simulink model "xdot_obac_debug"  (Simulink 6.3)
settings: Solver=FixedStepDiscrete  StartTime=0.0  StopTime=0  RelTol=1e-3
undefined symbols (not defined in the file or in its folder): aero, bspan, cbar, constants, Frcs, MACH, MACH_mass_IC, obac_params, r_aero, r_prop, r_rcs, rcs_idx, Sref, throt_to_ff, tvc_idx
libraries: simulink x14, models x14, utility_lib x12, model_lib x3, aerospace x1
settings Model: LastModifiedBy=E700252  BufferReuse=off  StrictBusMsg=None
settings DataIOCC: ExternalInput=[0 xu]  InitialState=[]  LoadExternalInput=on  LoadInitialState=on  SaveOutput=off  SaveTime=off  SignalLoggingName=sigsOut
settings OptimizationCC: InlineParams=on  BufferReuse=off
settings DebuggingCC: SolverPrmCheckMsg=none
settings HardwareCC: TargetUnknown=on

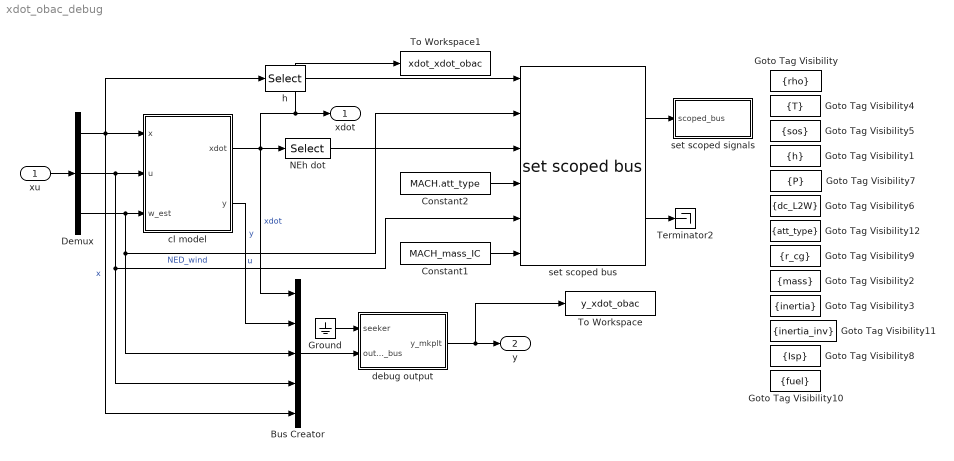
== system xdot_obac_debug ==
  xu : Inport
  Bus Creator : BusCreator  Inputs=5
  Constant1 : Constant  Value=MACH_mass_IC
  Constant2 : Constant  Value=MACH.att_type
  Demux : Demux  Outputs=[MACH.num_x MACH.num_u 3]
  Goto Tag Visibility : GotoTagVisibility  GotoTag=rho
  Goto Tag Visibility1 : GotoTagVisibility  GotoTag=h
  Goto Tag Visibility10 : GotoTagVisibility  GotoTag=fuel
  Goto Tag Visibility11 : GotoTagVisibility  GotoTag=inertia_inv
  Goto Tag Visibility12 : GotoTagVisibility  GotoTag=att_type
  Goto Tag Visibility2 : GotoTagVisibility  GotoTag=mass
  Goto Tag Visibility3 : GotoTagVisibility  GotoTag=inertia
  Goto Tag Visibility4 : GotoTagVisibility  GotoTag=T
  Goto Tag Visibility5 : GotoTagVisibility  GotoTag=sos
  Goto Tag Visibility6 : GotoTagVisibility  GotoTag=dc_L2W
  Goto Tag Visibility7 : GotoTagVisibility  GotoTag=P
  Goto Tag Visibility8 : GotoTagVisibility  GotoTag=Isp
  Goto Tag Visibility9 : GotoTagVisibility  GotoTag=r_cg
  Ground : Ground
  NEh dot : Selector  Elements=MACH.NEh_idx  InputPortWidth=obac_params.num_x
  Terminator2 : Terminator
  To Workspace : ToWorkspace  VariableName=y_xdot_obac  SampleTime=-1  SaveFormat=Array
  To Workspace1 : ToWorkspace  VariableName=xdot_xdot_obac  SampleTime=-1  SaveFormat=Array
  cl model : Subsystem  AncestorBlock=models/datcom-obac
  debug output : Subsystem
  h : Selector  Elements=MACH.NEh_idx(3)  InputPortWidth=obac_params.num_x
  set scoped bus : model_lib/set scoped bus  vehicle_params=obac_params
  set scoped signals : Subsystem  AncestorBlock=model_lib/set scoped signals
  xdot : Outport
  y : Outport  Port=2
  wires:
  Demux/1 -> cl model/1(x), h/1, Bus Creator/5  "x"
  Demux/2 -> cl model/2(u), set scoped bus/5, Bus Creator/4  "u"
  Demux/3 -> cl model/3(w_est), set scoped bus/2, Bus Creator/3  "NED_wind"
  xu/1 -> Demux/1
  cl model/1(xdot) -> NEh dot/1, Bus Creator/1, xdot/1, To Workspace1/1  "xdot"
  h/1 -> set scoped bus/1
  NEh dot/1 -> set scoped bus/3
  Constant2/1 -> set scoped bus/4
  set scoped bus/1 -> set scoped signals/1(scoped_bus)
  Constant1/1 -> set scoped bus/6
  set scoped bus/2 -> Terminator2/1
  debug output/1(y_mkplt) -> y/1, To Workspace/1
  Ground/1 -> debug output/1(seeker)
  Bus Creator/1 -> debug output/2(output_bus)
  cl model/2(y) -> Bus Creator/2  "y"

== system xdot_obac_debug/cl model ==
  x : Inport
  u : Inport  Port=2
  w_est : Inport  Port=3
  datcom-kernel : Subsystem  AncestorBlock=models/datcom-kernel  mask{vehicle_params=obac_params}
      mask prompts: vehicle_params "vehicle params"
      mask init:
      | paramnames = fieldnames(vehicle_params);
      | for i=1:length(paramnames)
      | 	eval([paramnames{i} '= vehicle_params.' paramnames{i} ';']);
      | end
  xdot : Outport
  y : Outport  Port=2
  wires:
  datcom-kernel/2(y) -> y/1
  datcom-kernel/1(xdot) -> xdot/1
  w_est/1 -> datcom-kernel/3(w_est)
  u/1 -> datcom-kernel/2(u)
  x/1 -> datcom-kernel/1(x)

== system xdot_obac_debug/debug output ==
  seeker : Inport
  output_bus : Inport  Port=2
  Bus Creator1 : BusCreator  Inputs=7
  Bus Selector : BusSelector  OutputSignals=y.dircos,x,NED_wind
  Gain : Gain  SaturateOnIntegerOverflow=on
  angles : Subsystem
  order outputs as expected by mkplt : BusSelector  OutputSignals=output_bus.y.accels,output_bus.y.accels_cg,output_bus.y.dircos,uvw_rw,tilta;tiltb;cam,phi;theta;psi,mu;alpha;beta,mass,output_bus.y.aero_env,seeker  OutputAsBus=on
  uvw : Selector  Elements=MACH.uvw_idx  InputPortWidth=MACH.num_x
  y_mkplt : Outport
  wires:
  Bus Selector/2 -> uvw/1  "<x>"
  Bus Creator1/1 -> order outputs as expected by mkplt/1
  Bus Selector/3 -> angles/3(NED_wind)  "<NED_wind>"
  uvw/1 -> angles/2(uvw)
  Bus Selector/1 -> angles/1(dircos)  "<dircos>"
  seeker/1 -> Bus Creator1/7  "seeker"
  [mass] -> Bus Creator1/6  "mass"
  Gain/1 -> y_mkplt/1
  order outputs as expected by mkplt/1 -> Gain/1
  output_bus/1 -> Bus Creator1/1, Bus Selector/1  "output_bus"
  angles/3(phi;theta;psi) -> Bus Creator1/4  "phi;theta;psi"
  angles/2(tilta;tiltb;cam) -> Bus Creator1/3  "tilta;tiltb;cam"
  angles/1(uvw_rw) -> Bus Creator1/2  "uvw_rw"
  angles/4(mu;alpha;beta) -> Bus Creator1/5  "mu;alpha;beta"

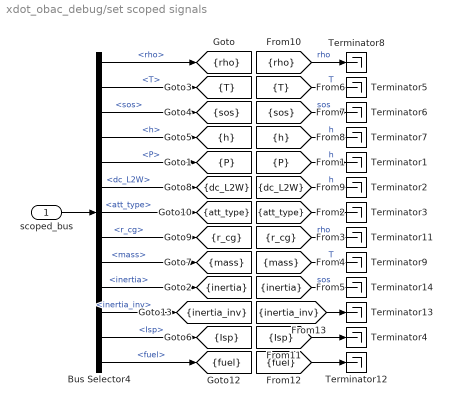
== system xdot_obac_debug/set scoped signals ==
  scoped_bus : Inport
  Bus Selector4 : BusSelector  OutputSignals=atmos_env.rho,atmos_env.T,atmos_env.sos,atmos_env.h,atmos_env.P,dc_L2W,att_type,mass_props.r_cg,mass_props.mass,mass_props.inertia,mass_props.inertia_inv,mass_props.Isp,mass_props.fuel
  Terminator{1..9,11..14} (13 alike) : Terminator
  tag scope: Isp=scoped, P=scoped, T=scoped, att_type=scoped, dc_L2W=scoped, fuel=scoped, h=scoped, inertia=scoped, inertia_inv=scoped, mass=scoped, r_cg=scoped, rho=scoped, sos=scoped
  wires:
  scoped_bus/1 -> Bus Selector4/1
  Bus Selector4/1 -> [rho]  "<rho>"
  Bus Selector4/2 -> [T]  "<T>"
  Bus Selector4/3 -> [sos]  "<sos>"
  Bus Selector4/4 -> [h]  "<h>"
  Bus Selector4/5 -> [P]  "<P>"
  Bus Selector4/6 -> [dc_L2W]  "<dc_L2W>"
  Bus Selector4/7 -> [att_type]  "<att_type>"
  Bus Selector4/8 -> [r_cg]  "<r_cg>"
  Bus Selector4/9 -> [mass]  "<mass>"
  Bus Selector4/10 -> [inertia]  "<inertia>"
  Bus Selector4/12 -> [Isp]  "<Isp>"
  [h] -> Terminator7/1  "h"
  [sos] -> Terminator6/1  "sos"
  [T] -> Terminator5/1  "T"
  [rho] -> Terminator8/1  "rho"
  [P] -> Terminator1/1  "h"
  [dc_L2W] -> Terminator2/1  "h"
  [att_type] -> Terminator3/1
  [r_cg] -> Terminator11/1  "rho"
  [mass] -> Terminator9/1  "T"
  [inertia] -> Terminator14/1  "sos"
  [Isp] -> Terminator4/1
  Bus Selector4/13 -> [fuel]  "<fuel>"
  [fuel] -> Terminator12/1
  [inertia_inv] -> Terminator13/1
  Bus Selector4/11 -> [inertia_inv]  "<inertia_inv>"

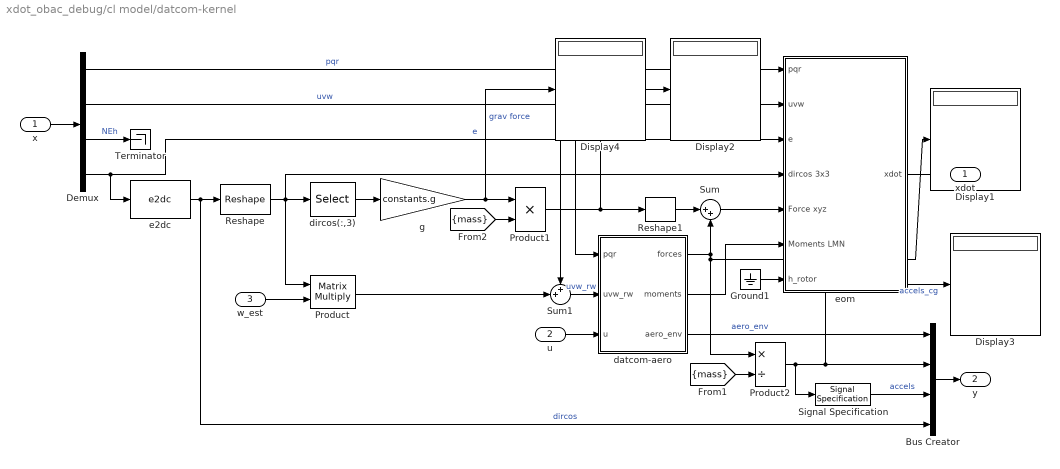
== system xdot_obac_debug/cl model/datcom-kernel ==
  x : Inport
  u : Inport  Port=2
  w_est : Inport  Port=3
  Bus Creator : BusCreator
  Demux : Demux  Outputs=[3 3 3 4]
  Display{1..4} (4 alike) : Display
  Ground1 : Ground
  Product : Product  Multiplication=Matrix(*)  SaturateOnIntegerOverflow=on
  Product1 : Product  RndMeth=Zero
  Product2 : Product  Inputs=*/  RndMeth=Zero
  Reshape : simulink/Math Operations/Reshape  OutputDimensionality=Customize  OutputDimensions=[3,3]
  Reshape1 : simulink/Math Operations/Reshape  OutputDimensionality=1-D array  OutputDimensions=[1,1]
  Signal Specification : SignalSpecification
  Sum : Sum  Inputs=|++  SaturateOnIntegerOverflow=on
  Sum1 : Sum  Inputs=++|  SaturateOnIntegerOverflow=on
  Terminator : Terminator
  datcom-aero : Subsystem  AncestorBlock=models/datcom-aero  mask{aero_params=aero}
      mask prompts: aero_params "aero params"
      mask init:
      | paramnames = fieldnames(aero_params);
      | for i=1:length(paramnames)
      | 	eval([paramnames{i} '= aero_params.' paramnames{i} ';']);
      | end
  dircos(:,3) : Selector  InputType=Matrix  Elements=[7:9]  Rows=-1  Columns=3  InputPortWidth=9
  e2dc : utility_lib/e2dc
  eom : Subsystem  AncestorBlock=model_lib/eom
  g : Gain  Gain=constants.g  SaturateOnIntegerOverflow=on
  xdot : Outport
  y : Outport  Port=2
  wires:
  Signal Specification/1 -> Bus Creator/3  "accels"
  Bus Creator/1 -> y/1
  [mass] -> Product2/2
  Product2/1 -> Signal Specification/1, Bus Creator/2, Display3/1  "accels_cg"
  x/1 -> Demux/1
  Demux/1 -> datcom-aero/1(pqr), eom/1(pqr)  "pqr"
  Demux/3 -> Terminator/1  "NEh"
  Demux/4 -> eom/3(e), e2dc/1  "e"
  Demux/2 -> eom/2(uvw), Sum1/1  "uvw"
  dircos(:,3)/1 -> g/1
  g/1 -> Product1/1, Display4/1  "grav force"
  eom/1(xdot) -> xdot/1
  e2dc/1 -> Bus Creator/4, Reshape/1  "dircos"
  u/1 -> datcom-aero/3(u)
  datcom-aero/1(forces) -> Sum/2, Product2/1, Display1/1
  Sum1/1 -> datcom-aero/2(uvw_rw)  "uvw_rw"
  w_est/1 -> Product/2
  Product/1 -> Sum1/2
  Sum/1 -> eom/5("Force xyz ")
  Reshape/1 -> eom/4(dircos 3x3), dircos(:,3)/1, Product/1
  Reshape1/1 -> Sum/1
  datcom-aero/2(moments) -> eom/6(Moments LMN)
  Ground1/1 -> eom/7(h_rotor)
  datcom-aero/3(aero_env) -> Bus Creator/1  "aero_env"
  Product1/1 -> Reshape1/1, Display2/1
  [mass] -> Product1/2

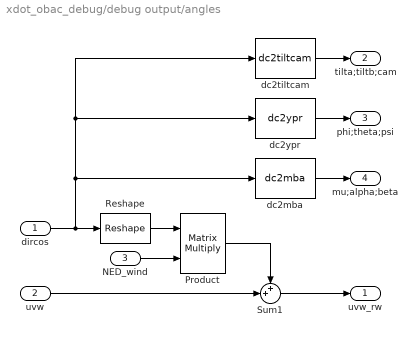
== system xdot_obac_debug/debug output/angles ==
  dircos : Inport
  uvw : Inport  Port=2
  NED_wind : Inport  Port=3
  Product : Product  Multiplication=Matrix(*)  SaturateOnIntegerOverflow=on
  Reshape : simulink/Math Operations/Reshape  OutputDimensionality=Customize  OutputDimensions=[3,3]
  Sum1 : Sum  Inputs=++|  SaturateOnIntegerOverflow=on
  dc2mba : utility_lib/dc2mba
  dc2tiltcam : utility_lib/dc2tiltcam
  dc2ypr : utility_lib/dc2ypr
  uvw_rw : Outport
  tilta;tiltb;cam : Outport  Port=2
  phi;theta;psi : Outport  Port=3
  mu;alpha;beta : Outport  Port=4
  wires:
  dircos/1 -> dc2mba/1, dc2tiltcam/1, dc2ypr/1, Reshape/1
  Reshape/1 -> Product/1
  dc2mba/1 -> mu;alpha;beta/1
  dc2tiltcam/1 -> tilta;tiltb;cam/1
  dc2ypr/1 -> phi;theta;psi/1
  Sum1/1 -> uvw_rw/1
  uvw/1 -> Sum1/2
  Product/1 -> Sum1/1
  NED_wind/1 -> Product/2

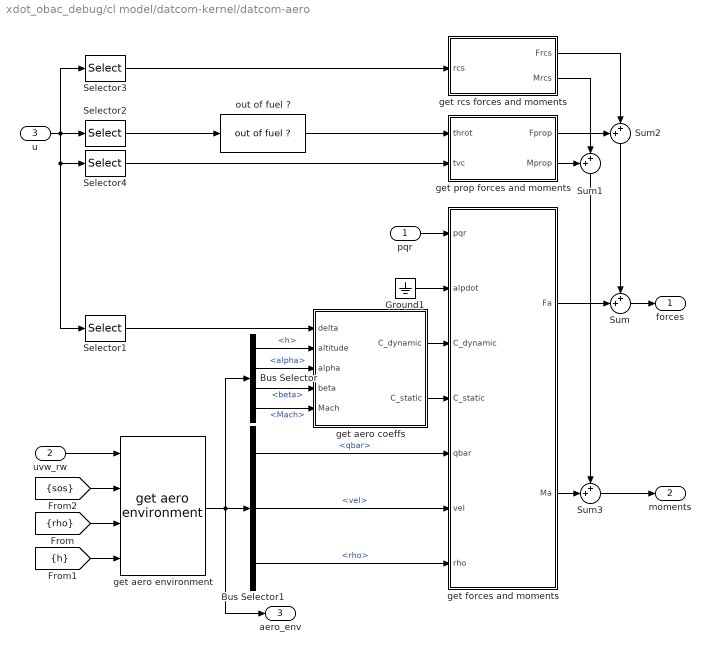
== system xdot_obac_debug/cl model/datcom-kernel/datcom-aero ==
  pqr : Inport
  uvw_rw : Inport  Port=2
  u : Inport  Port=3
  Bus Selector : BusSelector  OutputSignals=h,alpha,beta,Mach
  Bus Selector1 : BusSelector  OutputSignals=qbar,vel,rho
  Ground1 : Ground
  Selector1 : Selector  Elements=vane_idx  InputPortWidth=num_u
  Selector2 : Selector  Elements=throttle_idx  InputPortWidth=num_u
  Selector3 : Selector  Elements=[rcs_idx 1]  InputPortWidth=num_u
  Selector4 : Selector  Elements=tvc_idx  InputPortWidth=num_u
  Sum : Sum  Inputs=++|
  Sum1 : Sum  Orientation=down  Inputs=++|
  Sum2 : Sum  Orientation=down  Inputs=++|
  Sum3 : Sum  Inputs=++|
  get aero coeffs : Subsystem
  get aero environment : model_lib/get aero environment
  get forces and moments : Subsystem
  get prop forces and moments : Subsystem  AncestorBlock=model_lib/get prop forces and moments
  get rcs forces and moments : Subsystem
  out of fuel ? : model_lib/out of fuel ?
  forces : Outport
  moments : Outport  Port=2
  aero_env : Outport  Port=3
  wires:
  [rho] -> get aero environment/3
  pqr/1 -> get forces and moments/1(pqr)
  uvw_rw/1 -> get aero environment/1
  get aero coeffs/1(C_dynamic) -> get forces and moments/3(C_dynamic)
  get aero coeffs/2(C_static) -> get forces and moments/4(C_static)
  Ground1/1 -> get forces and moments/2(alpdot)
  get forces and moments/1(Fa) -> Sum/2
  Selector1/1 -> get aero coeffs/1(delta)
  [sos] -> get aero environment/2
  get aero environment/1 -> Bus Selector/1, Bus Selector1/1, aero_env/1
  Bus Selector/2 -> get aero coeffs/3(alpha)  "<alpha>"
  Bus Selector/3 -> get aero coeffs/4(beta)  "<beta>"
  Bus Selector/4 -> get aero coeffs/5(Mach)  "<Mach>"
  Bus Selector1/1 -> get forces and moments/5(qbar)  "<qbar>"
  Bus Selector1/2 -> get forces and moments/6(vel)  "<vel>"
  Bus Selector/1 -> get aero coeffs/2(altitude)  "<h>"
  [h] -> get aero environment/4
  Bus Selector1/3 -> get forces and moments/7(rho)  "<rho>"
  u/1 -> Selector2/1, Selector3/1, Selector1/1, Selector4/1
  Selector3/1 -> get rcs forces and moments/1(rcs)
  Sum/1 -> forces/1
  Sum3/1 -> moments/1
  get forces and moments/2(Ma) -> Sum3/2
  get rcs forces and moments/1(Frcs) -> Sum2/2
  get rcs forces and moments/2(Mrcs) -> Sum1/2
  get prop forces and moments/2(Mprop) -> Sum1/1
  get prop forces and moments/1(Fprop) -> Sum2/1
  Sum2/1 -> Sum/1
  Sum1/1 -> Sum3/1
  Selector2/1 -> out of fuel ?/1
  Selector4/1 -> get prop forces and moments/2(tvc)
  out of fuel ?/1 -> get prop forces and moments/1(throt)

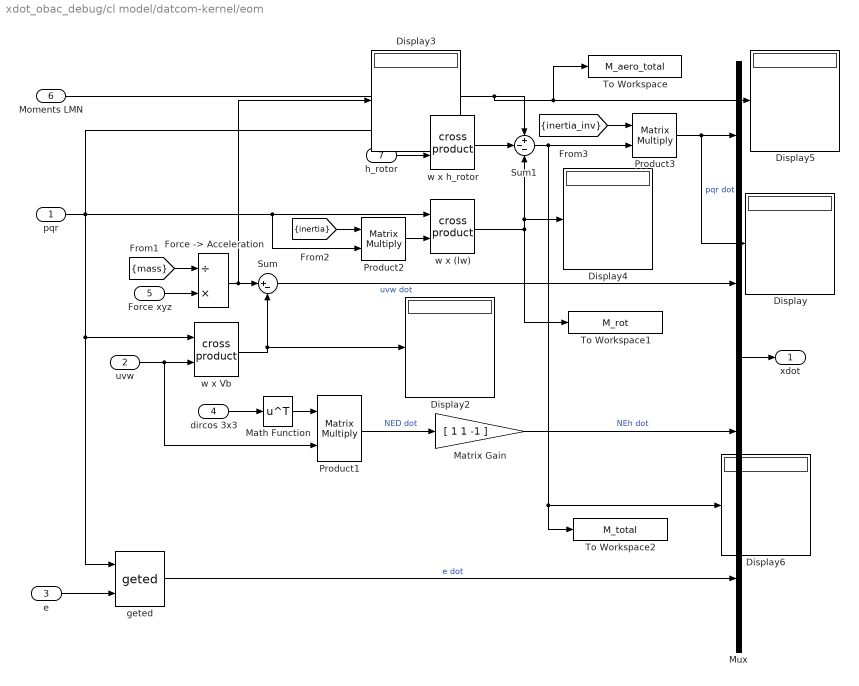
== system xdot_obac_debug/cl model/datcom-kernel/eom ==
  pqr : Inport
  uvw : Inport  Port=2
  e : Inport  Port=3
  dircos 3x3 : Inport  Port=4
  "Force xyz " : Inport  Port=5
  Moments LMN : Inport  Port=6
  h_rotor : Inport  Port=7
  Display{,2..6} (6 alike) : Display
  "Force -> Acceleration" : Product  Inputs=/*  RndMeth=Zero
  Math Function : Math  Operator=transpose  SaturateOnIntegerOverflow=on
  Matrix Gain : Gain  Gain=[ 1 1 -1 ]  SaturateOnIntegerOverflow=on
  Mux : Mux
  Product1 : Product  Multiplication=Matrix(*)  SaturateOnIntegerOverflow=on  InputSameDT=on
  Product2 : Product  Multiplication=Matrix(*)  RndMeth=Zero
  Product3 : Product  Multiplication=Matrix(*)  RndMeth=Zero
  Sum : Sum  Inputs=|+-  SaturateOnIntegerOverflow=on
  Sum1 : Sum  Inputs=+--  SaturateOnIntegerOverflow=on
  To Workspace : ToWorkspace  VariableName=M_aero_total  SampleTime=-1  SaveFormat=Array
  To Workspace1 : ToWorkspace  VariableName=M_rot  SampleTime=-1  SaveFormat=Array
  To Workspace2 : ToWorkspace  VariableName=M_total  SampleTime=-1  SaveFormat=Array
  geted : utility_lib/geted
  w x (lw) : utility_lib/cross product
  w x Vb : utility_lib/cross product
  w x h_rotor : utility_lib/cross product
  xdot : Outport
  wires:
  [inertia_inv] -> Product3/1
  [mass] -> "Force -> Acceleration"/1
  [inertia] -> Product2/1
  w x h_rotor/1 -> Sum1/2
  w x (lw)/1 -> Sum1/3, Display4/1, To Workspace1/1
  h_rotor/1 -> w x h_rotor/2
  "Force -> Acceleration"/1 -> Sum/1, Display3/1
  Math Function/1 -> Product1/1
  Product1/1 -> Matrix Gain/1  "NED dot"
  Sum1/1 -> Product3/2, Display6/1, To Workspace2/1
  Moments LMN/1 -> Sum1/1, Display5/1, To Workspace/1
  Product2/1 -> w x (lw)/2
  Product3/1 -> Mux/1, Display/1  "pqr dot"
  pqr/1 -> w x h_rotor/1, w x (lw)/1, Product2/2, w x Vb/1, geted/1
  dircos 3x3/1 -> Math Function/1
  Matrix Gain/1 -> Mux/3  "NEh dot"
  Sum/1 -> Mux/2  "uvw dot"
  "Force xyz "/1 -> "Force -> Acceleration"/2
  w x Vb/1 -> Sum/2, Display2/1
  uvw/1 -> w x Vb/2, Product1/2
  e/1 -> geted/2
  geted/1 -> Mux/4  "e dot"
  Mux/1 -> xdot/1

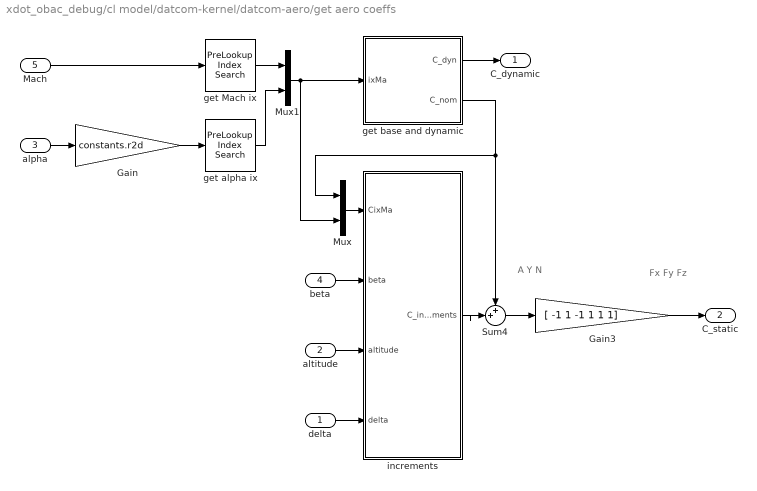
== system xdot_obac_debug/cl model/datcom-kernel/datcom-aero/get aero coeffs ==
  note: A
      | Y
      | N
  note: Fx
      | Fy
      | Fz
  delta : Inport
  altitude : Inport  Port=2
  alpha : Inport  Port=3
  beta : Inport  Port=4
  Mach : Inport  Port=5
  Gain : Gain  Gain=constants.r2d
  Gain3 : Gain  Gain=[ -1 1 -1 1 1 1]
  Mux : Mux  Inputs=2
  Mux1 : Mux  Inputs=2
  Sum4 : Sum  Inputs=++|
  get Mach ix : simulink/Lookup Tables/PreLookup Index Search  bpData=tbl_mach  searchMode=Binary Search  cacheBpFlag=off  outputFlag=off  IndexDataType=uint32  extrapMode=Linear Extrapolation  rangeErrorMode=None
  get alpha ix : simulink/Lookup Tables/PreLookup Index Search  bpData=tbl_alpha  searchMode=Binary Search  cacheBpFlag=off  outputFlag=off  IndexDataType=uint32  extrapMode=Linear Extrapolation  rangeErrorMode=None
  get base and dynamic : Subsystem
  increments : Subsystem
  C_dynamic : Outport
  C_static : Outport  Port=2
  wires:
  Mux1/1 -> get base and dynamic/1(ixMa), Mux/2
  get alpha ix/1 -> Mux1/2
  get Mach ix/1 -> Mux1/1
  alpha/1 -> Gain/1
  beta/1 -> increments/2(beta)
  delta/1 -> increments/4(delta)
  Mach/1 -> get Mach ix/1
  get base and dynamic/2(C_nom) -> Sum4/1, Mux/1
  Sum4/1 -> Gain3/1
  Mux/1 -> increments/1(CixMa)
  altitude/1 -> increments/3(altitude)
  increments/1(C_increments) -> Sum4/2
  get base and dynamic/1(C_dyn) -> C_dynamic/1
  Gain/1 -> get alpha ix/1
  Gain3/1 -> C_static/1

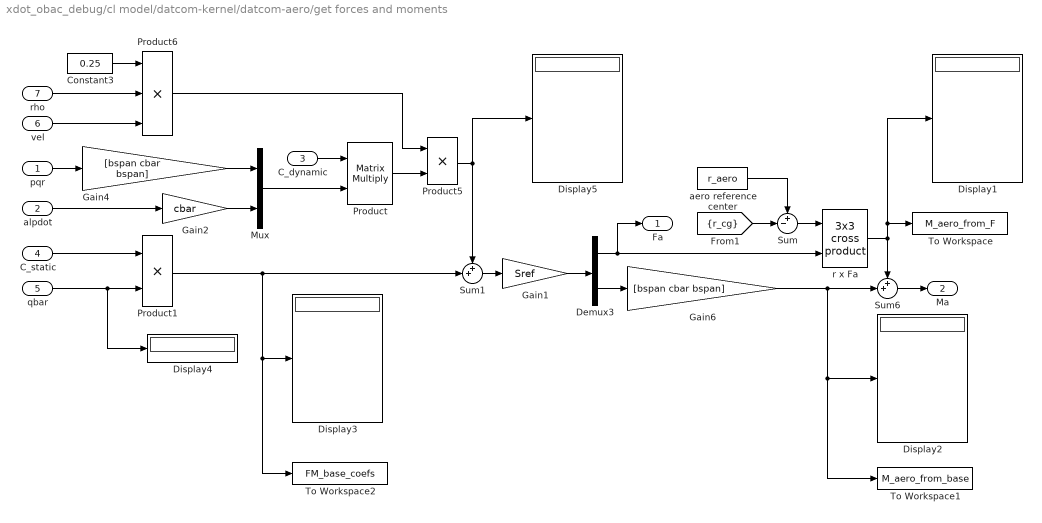
== system xdot_obac_debug/cl model/datcom-kernel/datcom-aero/get forces and moments ==
  pqr : Inport
  alpdot : Inport  Port=2
  C_dynamic : Inport  Port=3
  C_static : Inport  Port=4
  qbar : Inport  Port=5
  vel : Inport  Port=6
  rho : Inport  Port=7
  Constant3 : Constant  Value=0.25
  Demux3 : Demux  Outputs=2
  Display{1..5} (5 alike) : Display
  Gain1 : Gain  Gain=Sref
  Gain2 : Gain  Gain=cbar
  Gain4 : Gain  Gain=[bspan cbar bspan]
  Gain6 : Gain  Gain=[bspan cbar bspan]
  Mux : Mux  Inputs=2
  Product : Product  Multiplication=Matrix(*)  RndMeth=Zero
  Product1 : Product  RndMeth=Zero
  Product5 : Product  RndMeth=Zero
  Product6 : Product  Inputs=3  RndMeth=Zero
  Sum : Sum  Inputs=+-|
  Sum1 : Sum  Inputs=++|
  Sum6 : Sum  Inputs=++|
  To Workspace : ToWorkspace  VariableName=M_aero_from_F  SampleTime=-1  SaveFormat=Array
  To Workspace1 : ToWorkspace  VariableName=M_aero_from_base  SampleTime=-1  SaveFormat=Array
  To Workspace2 : ToWorkspace  VariableName=FM_base_coefs  SampleTime=-1  SaveFormat=Array
  aero reference center : Constant  Value=r_aero
  r x Fa : aerospace/Axes Transformations/3x3 cross product
  Fa : Outport
  Ma : Outport  Port=2
  wires:
  qbar/1 -> Product1/2, Display4/1
  C_static/1 -> Product1/1
  Gain1/1 -> Demux3/1
  Demux3/2 -> Gain6/1
  Demux3/1 -> r x Fa/2, Fa/1
  Sum1/1 -> Gain1/1
  Product/1 -> Product5/2
  Mux/1 -> Product/2
  Gain2/1 -> Mux/2
  Gain4/1 -> Mux/1
  alpdot/1 -> Gain2/1
  r x Fa/1 -> Sum6/1, Display1/1, To Workspace/1
  Sum6/1 -> Ma/1
  Constant3/1 -> Product6/1
  rho/1 -> Product6/2
  vel/1 -> Product6/3
  Product6/1 -> Product5/1
  Product5/1 -> Sum1/1, Display5/1
  Product1/1 -> Sum1/2, Display3/1, To Workspace2/1
  C_dynamic/1 -> Product/1
  pqr/1 -> Gain4/1
  Gain6/1 -> Sum6/2, Display2/1, To Workspace1/1
  aero reference center/1 -> Sum/1
  [r_cg] -> Sum/2
  Sum/1 -> r x Fa/1

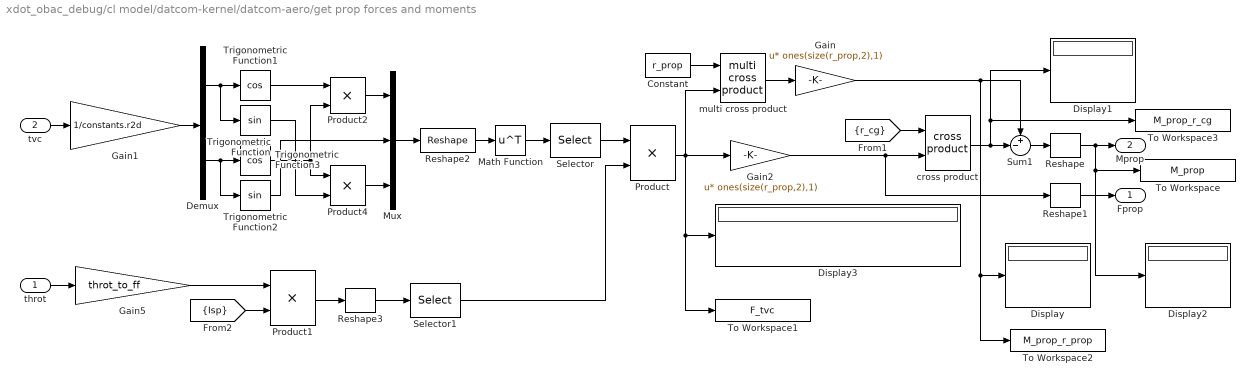
== system xdot_obac_debug/cl model/datcom-kernel/datcom-aero/get prop forces and moments ==
  throt : Inport
  tvc : Inport  Port=2
  Constant : Constant  Value=r_prop  VectorParams1D=off
  Demux : Demux  Outputs=2
  Display{,1..3} (4 alike) : Display
  Gain : Gain  Gain=ones(size(r_prop,2),1)  Multiplication=Matrix(u*K)
  Gain1 : Gain  Gain=1/constants.r2d
  Gain2 : Gain  Gain=ones(size(r_prop,2),1)  Multiplication=Matrix(u*K)
  Gain5 : Gain  Gain=throt_to_ff
  Math Function : Math  Operator=transpose  SaturateOnIntegerOverflow=on
  Mux : Mux  Inputs=3
  Product{,1..2,4} (4 alike) : Product  RndMeth=Zero
  Reshape : simulink/Math Operations/Reshape  OutputDimensionality=1-D array  OutputDimensions=[1,1]
  Reshape1 : simulink/Math Operations/Reshape  OutputDimensionality=1-D array  OutputDimensions=[1,1]
  Reshape2 : simulink/Math Operations/Reshape  OutputDimensionality=Customize  OutputDimensions=[length(tvc_idx)/2 3]
  Reshape3 : simulink/Math Operations/Reshape  OutputDimensionality=Row vector  OutputDimensions=[1,1]
  Selector : Selector  InputType=Matrix  Elements=[1 3]  Rows=-1  Columns=min(1:size(r_prop,2),length(tvc_idx)/2)  InputPortWidth=3
  Selector1 : Selector  InputType=Matrix  Elements=[1 3]  Rows=ones(1,size(r_prop,2))  Columns=-1  InputPortWidth=3
  Sum1 : Sum  Inputs=+-|
  To Workspace : ToWorkspace  VariableName=M_prop  SampleTime=-1  SaveFormat=Array
  To Workspace1 : ToWorkspace  VariableName=F_tvc  SampleTime=-1  SaveFormat=Array
  To Workspace2 : ToWorkspace  VariableName=M_prop_r_prop  SampleTime=-1  SaveFormat=Array
  To Workspace3 : ToWorkspace  VariableName=M_prop_r_cg  SampleTime=-1  SaveFormat=Array
  Trigonometric Function : Trigonometry
  Trigonometric Function1 : Trigonometry  Operator=cos
  Trigonometric Function2 : Trigonometry
  Trigonometric Function3 : Trigonometry  Operator=cos
  cross product : utility_lib/cross product
  multi cross product : utility_lib/multi cross product
  Fprop : Outport
  Mprop : Outport  Port=2
  wires:
  Reshape3/1 -> Selector1/1
  Selector1/1 -> Product/2
  Selector/1 -> Product/1
  Math Function/1 -> Selector/1
  Reshape2/1 -> Math Function/1
  Reshape1/1 -> Fprop/1
  Reshape/1 -> Mprop/1, To Workspace/1, Display2/1
  Sum1/1 -> Reshape/1
  cross product/1 -> Sum1/2, Display1/1, To Workspace3/1
  Gain/1 -> Sum1/1, Display/1, To Workspace2/1
  multi cross product/1 -> Gain/1
  Gain2/1 -> cross product/2, Reshape1/1
  [r_cg] -> cross product/1
  Product/1 -> multi cross product/2, Gain2/1, Display3/1, To Workspace1/1
  Constant/1 -> multi cross product/1
  tvc/1 -> Gain1/1
  Demux/1 -> Trigonometric Function1/1, Trigonometric Function/1
  Demux/2 -> Trigonometric Function3/1, Trigonometric Function2/1
  Product4/1 -> Mux/3
  Trigonometric Function3/1 -> Product2/2, Product4/1
  throt/1 -> Gain5/1
  Gain1/1 -> Demux/1
  Product2/1 -> Mux/1
  Trigonometric Function1/1 -> Product2/1
  Trigonometric Function/1 -> Product4/2
  Trigonometric Function2/1 -> Mux/2
  [Isp] -> Product1/2
  Gain5/1 -> Product1/1
  Mux/1 -> Reshape2/1
  Product1/1 -> Reshape3/1

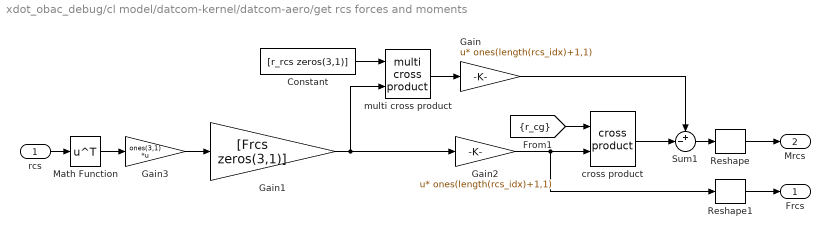
== system xdot_obac_debug/cl model/datcom-kernel/datcom-aero/get rcs forces and moments ==
  rcs : Inport
  Constant : Constant  Value=[r_rcs zeros(3,1)]  VectorParams1D=off
  Gain : Gain  Gain=ones(length(rcs_idx)+1,1)  Multiplication=Matrix(u*K)
  Gain1 : Gain  Gain=[Frcs zeros(3,1)]  SaturateOnIntegerOverflow=on
  Gain2 : Gain  Gain=ones(length(rcs_idx)+1,1)  Multiplication=Matrix(u*K)
  Gain3 : Gain  Gain=ones(3,1)  Multiplication=Matrix(K*u)
  Math Function : Math  Operator=transpose  SaturateOnIntegerOverflow=on
  Reshape : simulink/Math Operations/Reshape  OutputDimensionality=1-D array  OutputDimensions=[1,1]
  Reshape1 : simulink/Math Operations/Reshape  OutputDimensionality=1-D array  OutputDimensions=[1,1]
  Sum1 : Sum  Inputs=+-|
  cross product : utility_lib/cross product
  multi cross product : utility_lib/multi cross product
  Frcs : Outport
  Mrcs : Outport  Port=2
  wires:
  Constant/1 -> multi cross product/1
  Gain1/1 -> multi cross product/2, Gain2/1
  [r_cg] -> cross product/1
  Gain2/1 -> cross product/2, Reshape1/1
  multi cross product/1 -> Gain/1
  Gain/1 -> Sum1/1
  cross product/1 -> Sum1/2
  Sum1/1 -> Reshape/1
  rcs/1 -> Math Function/1
  Gain3/1 -> Gain1/1
  Math Function/1 -> Gain3/1
  Reshape/1 -> Mrcs/1
  Reshape1/1 -> Frcs/1

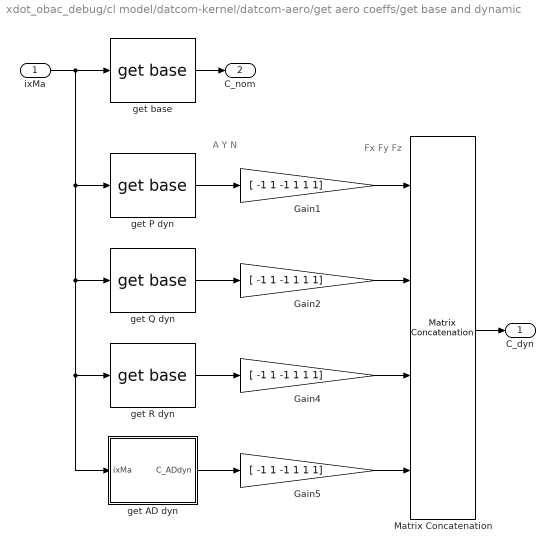
== system xdot_obac_debug/cl model/datcom-kernel/datcom-aero/get aero coeffs/get base and dynamic ==
  note: Fx
      | Fy
      | Fz
  note: A
      | Y
      | N
  ixMa : Inport
  Gain{1..2,4..5} (4 alike) : Gain  Gain=[ -1 1 -1 1 1 1]
  Matrix Concatenation : simulink/Math Operations/Matrix Concatenation  numInports=4  catMethod=Horizontal
  get AD dyn : Subsystem
  get P dyn : models/get base  delta_name='P'  aero=aero
  get Q dyn : models/get base  delta_name='Q'  aero=aero
  get R dyn : models/get base  delta_name='R'  aero=aero
  get base : models/get base  delta_name='nom'  aero=aero
  C_dyn : Outport
  C_nom : Outport  Port=2
  wires:
  Matrix Concatenation/1 -> C_dyn/1
  Gain5/1 -> Matrix Concatenation/4
  Gain4/1 -> Matrix Concatenation/3
  Gain2/1 -> Matrix Concatenation/2
  Gain1/1 -> Matrix Concatenation/1
  get AD dyn/1(C_ADdyn) -> Gain5/1
  get R dyn/1 -> Gain4/1
  get Q dyn/1 -> Gain2/1
  get P dyn/1 -> Gain1/1
  get base/1 -> C_nom/1
  ixMa/1 -> get base/1, get P dyn/1, get Q dyn/1, get R dyn/1, get AD dyn/1(ixMa)

== system xdot_obac_debug/cl model/datcom-kernel/datcom-aero/get aero coeffs/increments ==
  CixMa : Inport
  beta : Inport  Port=2
  altitude : Inport  Port=3
  delta : Inport  Port=4
  Gain : Gain  Gain=constants.r2d
  Sum : Sum  Inputs=+++
  get increment alt : models/get increment  delta_name='alt'  aero=aero
  get increment beta : models/get increment  delta_name='beta'  aero=aero
  surfaces : Subsystem
  C_increments : Outport
  wires:
  get increment alt/1 -> Sum/2
  beta/1 -> Gain/1
  get increment beta/1 -> Sum/1
  surfaces/1(C_surfaces) -> Sum/3
  Sum/1 -> C_increments/1
  altitude/1 -> get increment alt/2
  CixMa/1 -> get increment beta/1, get increment alt/1, surfaces/1(CixMa)
  delta/1 -> surfaces/2(delta)
  Gain/1 -> get increment beta/2

== system xdot_obac_debug/cl model/datcom-kernel/datcom-aero/get aero coeffs/get base and dynamic/get AD dyn ==
  ixMa : Inport
  CN TLU : simulink/Lookup Tables/Interpolation (n-D) using PreLookup  numDimsPopupSelect=2  explicitNumDims=2  table=tbl_CN_AD  interpMethod=Linear  extrapMethod=Linear  rangeErrorMode=None  NumSelectionDims=0
  Cm TLU : simulink/Lookup Tables/Interpolation (n-D) using PreLookup  numDimsPopupSelect=2  explicitNumDims=2  table=tbl_Cm_AD  interpMethod=Linear  extrapMethod=Linear  rangeErrorMode=None  NumSelectionDims=0
  Demux : Demux  Outputs=2
  Ground{,1..3} (4 alike) : Ground
  Mux : Mux  Inputs=6
  C_ADdyn : Outport
  wires:
  Ground2/1 -> Mux/4
  ixMa/1 -> Demux/1
  Cm TLU/1 -> Mux/5
  Ground3/1 -> Mux/6
  Ground1/1 -> Mux/2
  Ground/1 -> Mux/1
  CN TLU/1 -> Mux/3
  Mux/1 -> C_ADdyn/1
  Demux/2 -> CN TLU/2, Cm TLU/2
  Demux/1 -> CN TLU/1, Cm TLU/1

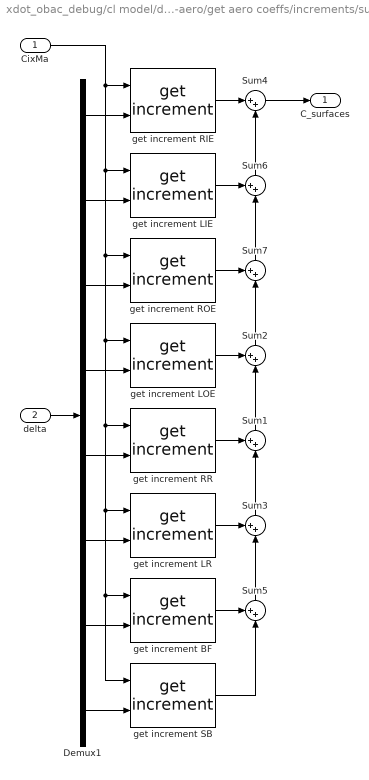
== system xdot_obac_debug/cl model/datcom-kernel/datcom-aero/get aero coeffs/increments/surfaces ==
  CixMa : Inport
  delta : Inport  Port=2
  Demux1 : Demux  Outputs=8
  Sum{1..3,5..7} (6 alike) : Sum  Orientation=up  Inputs=++|
  Sum4 : Sum  Inputs=|++
  get increment BF : models/get increment  delta_name='BF'  aero=aero
  get increment LIE : models/get increment  delta_name='LIE'  aero=aero
  get increment LOE : models/get increment  delta_name='LOE'  aero=aero
  get increment LR : models/get increment  delta_name='LR'  aero=aero
  get increment RIE : models/get increment  delta_name='RIE'  aero=aero
  get increment ROE : models/get increment  delta_name='ROE'  aero=aero
  get increment RR : models/get increment  delta_name='RR'  aero=aero
  get increment SB : models/get increment  delta_name='SB'  aero=aero
  C_surfaces : Outport
  wires:
  Sum7/1 -> Sum6/2
  get increment ROE/1 -> Sum7/1
  Sum6/1 -> Sum4/2
  delta/1 -> Demux1/1
  get increment RIE/1 -> Sum4/1
  Sum4/1 -> C_surfaces/1
  Demux1/1 -> get increment RIE/2
  Demux1/2 -> get increment LIE/2
  Demux1/3 -> get increment ROE/2
  Demux1/4 -> get increment LOE/2
  CixMa/1 -> get increment RIE/1, get increment LIE/1, get increment ROE/1, get increment LOE/1, get increment RR/1, get increment LR/1, get increment BF/1, get increment SB/1
  get increment LIE/1 -> Sum6/1
  Demux1/6 -> get increment LR/2
  Demux1/5 -> get increment RR/2
  get increment RR/1 -> Sum1/1
  get increment LOE/1 -> Sum2/1
  Sum2/1 -> Sum7/2
  Sum1/1 -> Sum2/2
  Demux1/7 -> get increment BF/2
  get increment LR/1 -> Sum3/1
  Sum3/1 -> Sum1/2
  Demux1/8 -> get increment SB/2
  get increment BF/1 -> Sum5/1
  Sum5/1 -> Sum3/2
  get increment SB/1 -> Sum5/2
